simulink model "exampleStorage_type1"  (R2016b)
settings: Solver=ode45  StartTime=0.0  StopTime=3*3600-2  MaxStep=300  RelTol=1e-3  EnableMultiTasking=on
libraries: carnot x8, simulink x2
settings Model: Creator=drhf  LastModifiedBy=drhf
settings DataIOCC: LimitDataPoints=on  SaveFormat=Array
settings OptimizationCC: ExpressionDepthLimit=2147483647  LifeSpan=inf
settings DebuggingCC: UnderspecifiedInitializationDetection=Classic  MergeDetectMultiDrivingBlocksExec=none  SolverPrmCheckMsg=warning  StateNameClashWarn=warning  SFUnexpectedBacktrackingDiag=warning  SFNoUnconditionalDefaultTransitionDiag=warning  SFExecutionAtInitializationDiag=none
settings HardwareCC: ProdBitPerPointer=32  ProdBitPerSizeT=32  ProdBitPerPtrDiffT=32  ProdLargestAtomicFloat=None  ProdIntDivRoundTo=Undefined  ProdEndianess=Unspecified  ProdWordSize=32  ProdHWDeviceType=32-bit Generic
settings ModelReferenceCC: PropagateSignalLabelsOutOfModel=off
settings GRTTargetCC: TargetLangStandard=C89/C90 (ANSI)  GeneratePreprocessorConditionals=Disable all  CombineOutputUpdateFcns=off  GRTInterface=on
settings ConfigComp: CovMetricSettings=dw  CovHtmlReporting=on  CovSaveCumulativeToWorkspaceVar=on  CovSaveSingleToWorkspaceVar=on  CovExternalEMLEnable=off

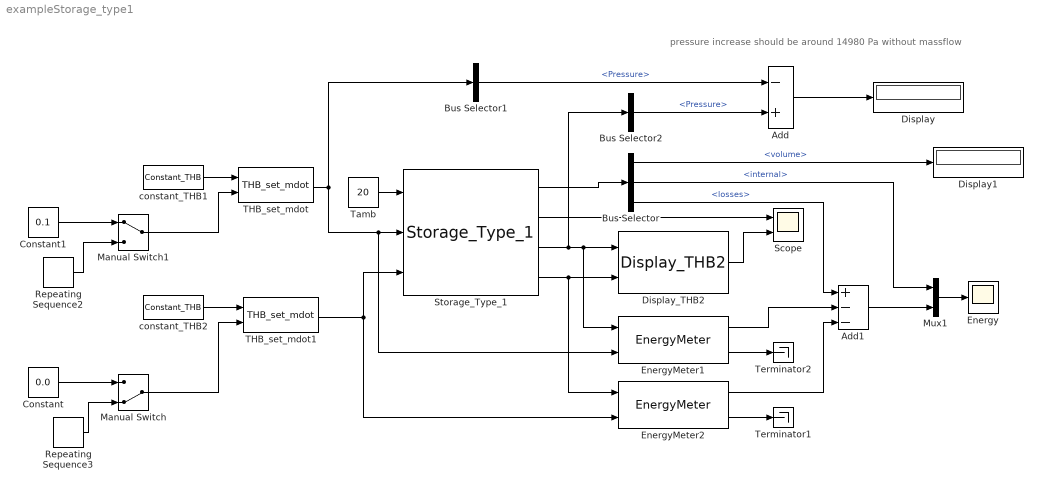
== system exampleStorage_type1 ==
  note: pressure increase should be around 14980 Pa without massflow
  Add : Sum  Inputs=-+
  Add1 : Sum  Inputs=+--
  Bus Selector : BusSelector  OutputSignals=volume,energy.internal,energy.losses
  Bus Selector1 : BusSelector  OutputSignals=Pressure
  Bus Selector2 : BusSelector  OutputSignals=Pressure
  Constant : Constant  Value=0.0
  Constant1 : Constant  Value=0.1
  Display : Display
  Display1 : Display
  Display_THB2 : carnot/Outputs/Display_THB2  t=off  m=on  p=off  id=off  mix=off  d=off
  Energy : Scope
  EnergyMeter1 : carnot/Control/EnergyMeter
  EnergyMeter2 : carnot/Control/EnergyMeter
  Manual Switch : ManualSwitch  CurrentSetting=0
  Manual Switch1 : ManualSwitch
  Mux1 : Mux  Inputs=2
  Repeating Sequence2 : simulink/Sources/Repeating Sequence  rep_seq_t=[ 0 3600 3600+eps(3600) 7200 7200+eps(7200) 10440 10440+eps(10440) 11160]  rep_seq_y=[ 0.12 0.12 0.15+0*eps(3600) 0.15 0.1+0*eps(7200) 0.1 0+0*eps(10440) 0]
  Repeating Sequence3 : simulink/Sources/Repeating Sequence  rep_seq_t=[ 0 3600 3600+eps(3600) 7200 7200+eps(7200) 10800]  rep_seq_y=[ 0.12 0.12 0.1+0*eps(3600) 0.1 0.15+0*eps(7200) 0.15]
  Scope : Scope  NumInputPorts=2
  Storage_Type_1 : carnot/Storage/Thermal/Storage_Type_1  uloss=1  ubot=1  utop=1  cond=1  volume=0.5  dia=0.6  pos=standing cylinder  h_in_chg=1  h_out_chg=0  dplin_chg=10  dpqua_chg=10  h_in=0  h_out=1  dplin=10  dpqua=10  t0=[10:5:55]  nodes=10  mpoints=10
  THB_set_mdot : carnot/Source/Simple/THB_set_mdot
  THB_set_mdot1 : carnot/Source/Simple/THB_set_mdot
  Tamb : Constant  Value=20
  Terminator1 : Terminator
  Terminator2 : Terminator
  constant_THB1 : carnot/Source/Simple/Constant_THB  t=55  mdot=0*100/3600  p=1e5  mID=Full Pressure Drop with Static Height  fluid=Water  mix=0  mix2=0  mix3=0  dia=0.02  hgt=0
  constant_THB2 : carnot/Source/Simple/Constant_THB  t=10  mdot=100/3600  p=1e5  mID=Full Pressure Drop with Static Height  fluid=Water  mix=0  mix2=0  mix3=0  dia=0.02  hgt=0
  wires:
  Bus Selector/2 -> Mux1/1  "<internal>"
  Tamb/1 -> Storage_Type_1/1
  THB_set_mdot/1 -> Bus Selector1/1, EnergyMeter1/2, Storage_Type_1/2
  THB_set_mdot1/1 -> Storage_Type_1/3, EnergyMeter2/2
  Storage_Type_1/1 -> Bus Selector/1
  Storage_Type_1/2 -> Scope/1
  Storage_Type_1/3 -> Bus Selector2/1, Display_THB2/1, EnergyMeter1/1
  Storage_Type_1/4 -> Display_THB2/2, EnergyMeter2/1
  Display_THB2/1 -> Scope/2
  Mux1/1 -> Energy/1
  EnergyMeter2/2 -> Terminator1/1
  constant_THB1/1 -> THB_set_mdot/1
  constant_THB2/1 -> THB_set_mdot1/1
  Manual Switch1/1 -> THB_set_mdot/2
  Manual Switch/1 -> THB_set_mdot1/2
  Add/1 -> Display/1
  Bus Selector1/1 -> Add/1  "<Pressure>"
  Bus Selector2/1 -> Add/2  "<Pressure>"
  Constant/1 -> Manual Switch/1
  Repeating Sequence3/1 -> Manual Switch/2
  Constant1/1 -> Manual Switch1/1
  Repeating Sequence2/1 -> Manual Switch1/2
  EnergyMeter1/2 -> Terminator2/1
  Add1/1 -> Mux1/2
  EnergyMeter2/1 -> Add1/3
  EnergyMeter1/1 -> Add1/2
  Bus Selector/3 -> Add1/1  "<losses>"
  Bus Selector/1 -> Display1/1  "<volume>"
